simulink model "Assignment1_final"  (R2021a)
settings: Solver=FixedStepAuto  StartTime=0.0  StopTime=10.0  FixedStep=1e-3  RelTol=1e-3  EnableMultiTasking=on
undefined symbols (not defined in the file): a, b, c, D0, D1, D10, D11, D12, D13, D2, D3, D4, D5, D6, D7, D8, D9, magnitude, PTA0, PTA1, PTA2, PTB23, PTB9, PTC16, PTC17, PTC2, PTC3, PTC4, PTD0, PTD1, PTD2, PTD3
libraries: frdmk64flib x19, dspstat3 x1, hdlsllib x1
settings Model: EnablePacing=on  PacingRate=0.250000  ExtModeTrigDuration=5  Creator=Arun Mistry  LastModifiedBy=jesti
settings OptimizationCC: EnhancedBackFolding=on  PassReuseOutputArgsAs=Individual arguments  ZeroExternalMemoryAtStartup=off  ZeroInternalMemoryAtStartup=off  MaxStackSize=64  OptimizeBlockOrder=speed  DifferentSizesBufferReuse=on  OptimizationCustomize=off  EfficientTunableParamExpr=on
settings DebuggingCC: ParameterTunabilityLossMsg=error
settings HardwareCC: ProdBitPerPointer=32  ProdBitPerSizeT=32  ProdBitPerPtrDiffT=32  ProdLargestAtomicInteger=Long  ProdLargestAtomicFloat=Double  ProdWordSize=32  ProdHWDeviceType=ARM Compatible->ARM Cortex
settings SFSimCC: MATLABDynamicMemAlloc=off
settings RTWCC: SystemTargetFile=ert.tlc  HardwareBoard=NXP FRDM-K64F  TLCOptions="-aInlineSetEventsForThisBaseRateFcn=TLC_FALSE -aSuppressMultiTaskScheduler=TLC_FALSE  -aRateBasedStepFcn=0"  TemplateMakefile=ert_default_tmf  Toolchain=GNU Tools for ARM Embedded Processors
settings CodeAppCC: ForceParamTrailComments=on  IgnoreCustomStorageClasses=off  OperatorAnnotations=on  SimulinkDataObjDesc=on  SFDataObjDesc=on  InsertBlockDesc=on
settings ERTTargetCC: ExtModeTransport=4  ExtModeMexFile=sendToCommService

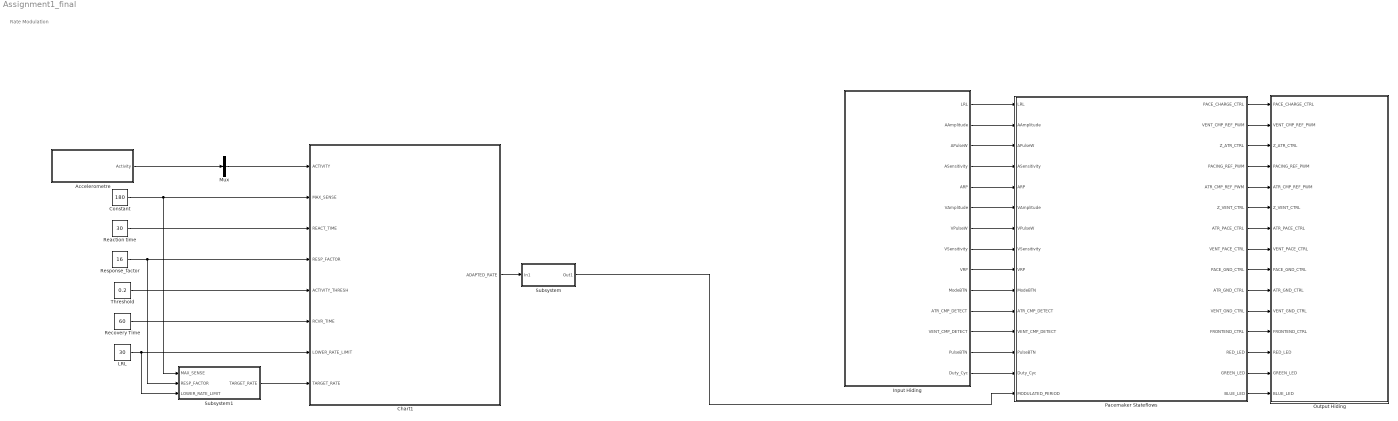
== system Assignment1_final ==
  note: Rate Modulation
  Accelerometre : Subsystem
  Chart1 : Stateflow chart  TreatAsAtomicUnit=on
  Constant : Constant  Value=180  OutDataTypeStr=uint16
  Input Hiding : Subsystem
  LRL : Constant  Value=30  OutDataTypeStr=uint16
  Mux : Mux  Inputs=1
  Output Hiding : Subsystem
  Pacemaker Stateflows : Stateflow chart  TreatAsAtomicUnit=on
      settings: PortSchema="{\"entries\":[{\"content\":{\"sides\":[{\"content\":{\"connectorIds\":[\"In1\",\"In2\",\"In3\",\"In4\",\"In5\",\"In6\",\"In7\",\"In8\",\"In9\",\"In10\",\"In11\",\"In12\",\"In13\",\"In15\",\"In14\"]},\"type\":\"ConnectorPlacement.EquallySpacedRectSide\",\"uuid\":\"73ec282f-bdc5-469f-8e6f-a94c3bdc9020\"},{\"content\":{\"connectorIds\":[\"Out1\",\"Out2\",\"Out3\",\"Out4\",\"Out5\",\"Out6\",\"Out7\",\"Out8\",\"Out9\",\"Out10\",\"Out11\",\"Out12\",\"Out13\",\"Out14\",\"Out15\"],\"side\":\"RIGHT\"},\"type\":\"ConnectorPlacement.EquallySpacedRectSide\",\"uuid\":\"8dd20006-a4c5-4baa-83a8-987332cd4bb4\"},{\"content\":{\"connectorIds\":[],\"side\":\"TOP\"},\"type\":\"ConnectorPlacement.EquallySpacedRectSide\",\"uuid\":\"22935e9b-efaa-43e1-8cc8-2e08fa14d9a6\"},{\"content\":{\"connectorIds\":[],\"side\":\"BOTTOM\"},\"type\":\"ConnectorPlacement.EquallySpacedRectSide\",\"uuid\":\"9851d334-d076-4ac0-89c9-77644970121a\"}]},\"type\":\"ConnectorPlacement.EquallySpacedConnector\",\"uuid\":\"2847227f-03fa-454f-95d6-41e472bd469d\"}],\"packageUris\":[\"http://schema.mathworks.com/mf0/Connector/R2020b\"],\"version\":\"1.0\"}"
  Reaction time : Constant  Value=30  OutDataTypeStr=uint16
  Recovery Time : Constant  Value=60  OutDataTypeStr=uint16
  Response_factor : Constant  Value=16  OutDataTypeStr=uint16
  Subsystem : Subsystem
  Subsystem1 : Subsystem
  Threshold : Constant  Value=0.2  OutDataTypeStr=double
  wires:
  Input Hiding/13(PulseBTN) -> Pacemaker Stateflows/13(PulseBTN)
  Pacemaker Stateflows/1(PACE_CHARGE_CTRL) -> Output Hiding/1(PACE_CHARGE_CTRL)
  Input Hiding/11(ATR_CMP_DETECT) -> Pacemaker Stateflows/11(ATR_CMP_DETECT)
  Input Hiding/7(VPulseW) -> Pacemaker Stateflows/7(VPulseW)
  Input Hiding/12(VENT_CMP_DETECT) -> Pacemaker Stateflows/12(VENT_CMP_DETECT)
  Pacemaker Stateflows/3(Z_ATR_CTRL) -> Output Hiding/3(Z_ATR_CTRL)
  Input Hiding/3(APulseW) -> Pacemaker Stateflows/3(APulseW)
  Pacemaker Stateflows/7(ATR_PACE_CTRL) -> Output Hiding/7(ATR_PACE_CTRL)
  Pacemaker Stateflows/10(ATR_GND_CTRL) -> Output Hiding/10(ATR_GND_CTRL)
  Input Hiding/10(ModeBTN) -> Pacemaker Stateflows/10(ModeBTN)
  Input Hiding/2(AAmplitude) -> Pacemaker Stateflows/2(AAmplitude)
  Input Hiding/6(VAmplitude) -> Pacemaker Stateflows/6(VAmplitude)
  Pacemaker Stateflows/6(Z_VENT_CTRL) -> Output Hiding/6(Z_VENT_CTRL)
  Pacemaker Stateflows/4(PACING_REF_PWM) -> Output Hiding/4(PACING_REF_PWM)
  Pacemaker Stateflows/11(VENT_GND_CTRL) -> Output Hiding/11(VENT_GND_CTRL)
  Pacemaker Stateflows/9(PACE_GND_CTRL) -> Output Hiding/9(PACE_GND_CTRL)
  Pacemaker Stateflows/8(VENT_PACE_CTRL) -> Output Hiding/8(VENT_PACE_CTRL)
  Input Hiding/1(LRL) -> Pacemaker Stateflows/1(LRL)
  Pacemaker Stateflows/15(BLUE_LED) -> Output Hiding/15(BLUE_LED)
  Input Hiding/4(ASensitivity) -> Pacemaker Stateflows/4(ASensitivity)
  Pacemaker Stateflows/12(FRONTEND_CTRL) -> Output Hiding/12(FRONTEND_CTRL)
  Input Hiding/9(VRP) -> Pacemaker Stateflows/9(VRP)
  Input Hiding/8(VSensitivity) -> Pacemaker Stateflows/8(VSensitivity)
  Input Hiding/5(ARP) -> Pacemaker Stateflows/5(ARP)
  Pacemaker Stateflows/14(GREEN_LED) -> Output Hiding/14(GREEN_LED)
  Pacemaker Stateflows/13(RED_LED) -> Output Hiding/13(RED_LED)
  Pacemaker Stateflows/5(ATR_CMP_REF_PWM) -> Output Hiding/5(ATR_CMP_REF_PWM)
  Pacemaker Stateflows/2(VENT_CMP_REF_PWM) -> Output Hiding/2(VENT_CMP_REF_PWM)
  Input Hiding/14(Duty_Cyc) -> Pacemaker Stateflows/15(Duty_Cyc)
  LRL/1 -> Chart1/7(LOWER_RATE_LIMIT), Subsystem1/3(LOWER_RATE_LIMIT)
  Chart1/1(ADAPTED_RATE) -> Subsystem/1(In1)
  Subsystem1/1(TARGET_RATE) -> Chart1/8(TARGET_RATE)
  Mux/1 -> Chart1/1(ACTIVITY)
  Recovery Time/1 -> Chart1/6(RCVR_TIME)
  Constant/1 -> Subsystem1/1(MAX_SENSE), Chart1/2(MAX_SENSE)
  Reaction time/1 -> Chart1/3(REACT_TIME)
  Response_factor/1 -> Subsystem1/2(RESP_FACTOR), Chart1/4(RESP_FACTOR)
  Accelerometre/1(Activity) -> Mux/1
  Threshold/1 -> Chart1/5(ACTIVITY_THRESH)
  Subsystem/1(Out1) -> Pacemaker Stateflows/14(MODULATED_PERIOD)

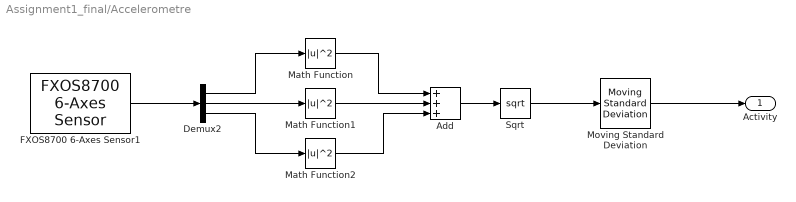
== system Assignment1_final/Accelerometre ==
  Add : Sum  Inputs=+++
  Demux2 : Demux  Outputs=3
  FXOS8700 6-Axes Sensor1 : frdmk64flib/FXOS8700 6-Axes Sensor  Activesensor=Accelerometer only  ODR=800Hz  HybridODR=400Hz  Accelfullrange=-4g to +4g  SampleTime=-1
  Math Function : Math  Operator=magnitude^2  SignedPower=on  OutDataTypeStr=double  SaturateOnIntegerOverflow=on
  Math Function1 : Math  Operator=magnitude^2  SignedPower=on  OutDataTypeStr=double  SaturateOnIntegerOverflow=on
  Math Function2 : Math  Operator=magnitude^2  SignedPower=on  OutDataTypeStr=double  SaturateOnIntegerOverflow=on
  Moving Standard Deviation : dspstat3/Moving Standard Deviation  Method=Sliding window  ForgettingFactorPort=off  SpecifyWindowLength=on  WindowLength=128  ForgettingFactor=0.9  SimulateUsing=Code generation
      settings: SourceProductBaseCode=DS
  Sqrt : Sqrt  SaturateOnIntegerOverflow=on
  Activity : Outport  SourceOfInitialOutputValue=Input signal
  wires:
  Sqrt/1 -> Moving Standard Deviation/1
  FXOS8700 6-Axes Sensor1/1 -> Demux2/1
  Math Function/1 -> Add/1
  Add/1 -> Sqrt/1
  Math Function2/1 -> Add/3
  Demux2/2 -> Math Function1/1
  Math Function1/1 -> Add/2
  Demux2/1 -> Math Function/1
  Demux2/3 -> Math Function2/1
  Moving Standard Deviation/1 -> Activity/1

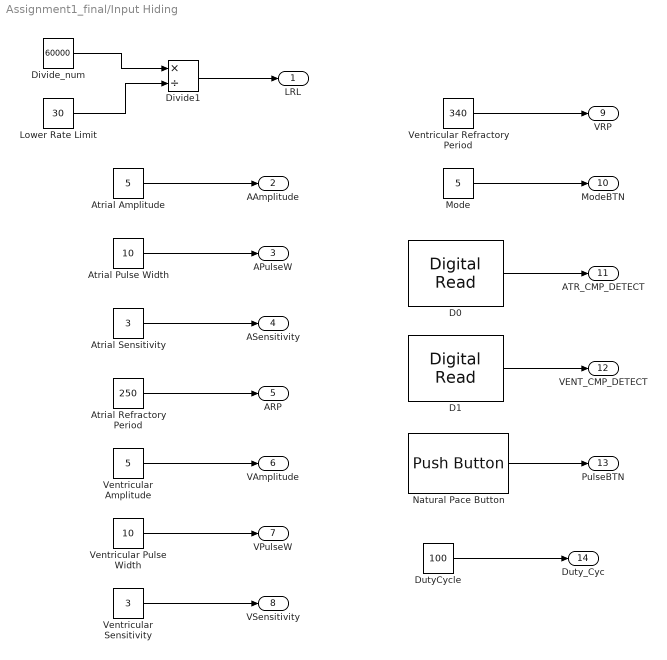
== system Assignment1_final/Input Hiding ==
  Atrial Amplitude : Constant  Value=5  OutDataTypeStr=uint16
  Atrial Pulse Width : Constant  Value=10  OutDataTypeStr=uint16
  Atrial Refractory Period : Constant  Value=250  OutDataTypeStr=uint16
  Atrial Sensitivity : Constant  Value=3  OutDataTypeStr=uint16
  D0 : frdmk64flib/Digital Read  Whichpin=PTC16 (D0)  SampleTime=-1
  D1 : frdmk64flib/Digital Read  Whichpin=PTC17 (D1)  SampleTime=-1
  Divide1 : Product  Inputs=*/  OutDataTypeStr=uint16  RndMeth=Round
  Divide_num : Constant  Value=60000  OutDataTypeStr=uint16
  DutyCycle : Constant  Value=100  OutDataTypeStr=uint16
  Lower Rate Limit : Constant  Value=30  OutDataTypeStr=uint16
  Mode : Constant  Value=5  OutDataTypeStr=uint16
  Natural Pace Button : frdmk64flib/Push Button  Whichswitch=SW3  SampleTime1=-1
  Ventricular Amplitude : Constant  Value=5  OutDataTypeStr=uint16
  Ventricular Pulse Width : Constant  Value=10  OutDataTypeStr=uint16
  Ventricular Refractory Period : Constant  Value=340  OutDataTypeStr=uint16
  Ventricular Sensitivity : Constant  Value=3  OutDataTypeStr=uint16
  LRL : Outport  OutDataTypeStr=uint16
  AAmplitude : Outport  Port=2  OutDataTypeStr=uint16
  APulseW : Outport  Port=3  OutDataTypeStr=uint16
  ASensitivity : Outport  Port=4  OutDataTypeStr=uint16
  ARP : Outport  Port=5  OutDataTypeStr=uint16
  VAmplitude : Outport  Port=6  OutDataTypeStr=uint16
  VPulseW : Outport  Port=7  OutDataTypeStr=uint16
  VSensitivity : Outport  Port=8  OutDataTypeStr=uint16
  VRP : Outport  Port=9  OutDataTypeStr=uint16
  ModeBTN : Outport  Port=10  OutDataTypeStr=uint16
  ATR_CMP_DETECT : Outport  Port=11  OutDataTypeStr=boolean
  VENT_CMP_DETECT : Outport  Port=12  OutDataTypeStr=boolean
  PulseBTN : Outport  Port=13  OutDataTypeStr=boolean
  Duty_Cyc : Outport  Port=14  OutDataTypeStr=uint16
  wires:
  Atrial Amplitude/1 -> AAmplitude/1
  Ventricular Amplitude/1 -> VAmplitude/1
  Atrial Pulse Width/1 -> APulseW/1
  Ventricular Pulse Width/1 -> VPulseW/1
  Atrial Sensitivity/1 -> ASensitivity/1
  Ventricular Sensitivity/1 -> VSensitivity/1
  Ventricular Refractory Period/1 -> VRP/1
  Atrial Refractory Period/1 -> ARP/1
  D1/1 -> VENT_CMP_DETECT/1
  D0/1 -> ATR_CMP_DETECT/1
  Natural Pace Button/1 -> PulseBTN/1
  Mode/1 -> ModeBTN/1
  DutyCycle/1 -> Duty_Cyc/1
  Lower Rate Limit/1 -> Divide1/2
  Divide_num/1 -> Divide1/1
  Divide1/1 -> LRL/1

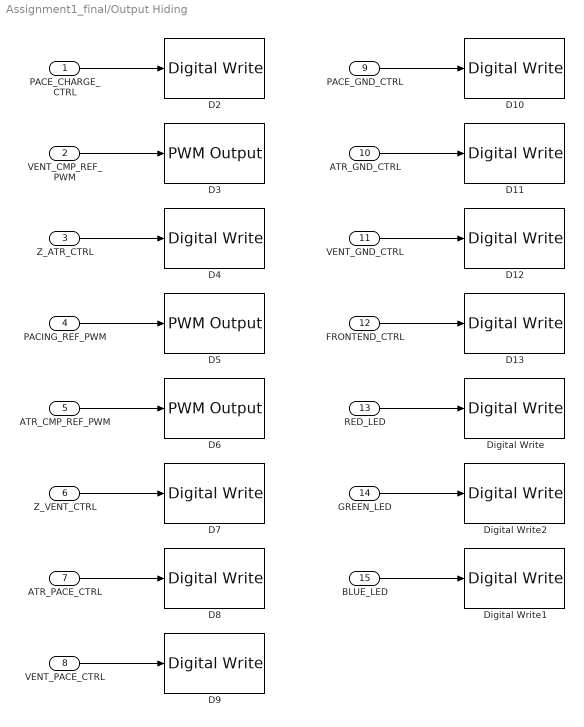
== system Assignment1_final/Output Hiding ==
  PACE_CHARGE_CTRL : Inport  OutDataTypeStr=uint16
  VENT_CMP_REF_PWM : Inport  Port=2  OutDataTypeStr=uint16
  Z_ATR_CTRL : Inport  Port=3  OutDataTypeStr=uint16
  PACING_REF_PWM : Inport  Port=4  OutDataTypeStr=uint16
  ATR_CMP_REF_PWM : Inport  Port=5  OutDataTypeStr=uint16
  Z_VENT_CTRL : Inport  Port=6  OutDataTypeStr=uint16
  ATR_PACE_CTRL : Inport  Port=7  OutDataTypeStr=uint16
  VENT_PACE_CTRL : Inport  Port=8  OutDataTypeStr=uint16
  PACE_GND_CTRL : Inport  Port=9  OutDataTypeStr=uint16
  ATR_GND_CTRL : Inport  Port=10  OutDataTypeStr=uint16
  VENT_GND_CTRL : Inport  Port=11  OutDataTypeStr=uint16
  FRONTEND_CTRL : Inport  Port=12  OutDataTypeStr=uint16
  RED_LED : Inport  Port=13  OutDataTypeStr=uint16
  GREEN_LED : Inport  Port=14  OutDataTypeStr=uint16
  BLUE_LED : Inport  Port=15  OutDataTypeStr=uint16
  D10 : frdmk64flib/Digital Write  Whichpin=PTD0 (D10)
  D11 : frdmk64flib/Digital Write  Whichpin=PTD2 (D11)
  D12 : frdmk64flib/Digital Write  Whichpin=PTD3 (D12)
  D13 : frdmk64flib/Digital Write  Whichpin=PTD1 (D13)
  D2 : frdmk64flib/Digital Write  Whichpin=PTB9 (D2)
  D3 : frdmk64flib/PWM Output  Whichpin=PTA1 (D3)  InitialFrequency=2000  InitialDutyCycle=100
  D4 : frdmk64flib/Digital Write  Whichpin=PTB23 (D4)
  D5 : frdmk64flib/PWM Output  Whichpin=PTA2 (D5)  InitialFrequency=2000  InitialDutyCycle=100
  D6 : frdmk64flib/PWM Output  Whichpin=PTC2 (D6)  InitialFrequency=2000  InitialDutyCycle=100
  D7 : frdmk64flib/Digital Write  Whichpin=PTC3 (D7)
  "D8 " : frdmk64flib/Digital Write  Whichpin=PTA0 (D8)
  D9 : frdmk64flib/Digital Write  Whichpin=PTC4 (D9)
  Digital Write : frdmk64flib/Digital Write  Whichpin=RED_LED
  Digital Write1 : frdmk64flib/Digital Write  Whichpin=BLUE_LED
  Digital Write2 : frdmk64flib/Digital Write  Whichpin=GREEN_LED
  wires:
  VENT_PACE_CTRL/1 -> D9/1
  ATR_CMP_REF_PWM/1 -> D6/1
  PACE_GND_CTRL/1 -> D10/1
  VENT_CMP_REF_PWM/1 -> D3/1
  PACING_REF_PWM/1 -> D5/1
  ATR_GND_CTRL/1 -> D11/1
  ATR_PACE_CTRL/1 -> "D8 "/1
  PACE_CHARGE_CTRL/1 -> D2/1
  FRONTEND_CTRL/1 -> D13/1
  VENT_GND_CTRL/1 -> D12/1
  Z_ATR_CTRL/1 -> D4/1
  Z_VENT_CTRL/1 -> D7/1
  RED_LED/1 -> Digital Write/1
  BLUE_LED/1 -> Digital Write1/1
  GREEN_LED/1 -> Digital Write2/1

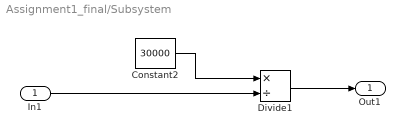
== system Assignment1_final/Subsystem ==
  In1 : Inport  OutDataTypeStr=uint16
  Constant2 : Constant  Value=30000  OutDataTypeStr=uint16
  Divide1 : Product  Inputs=*/  OutDataTypeStr=uint16
  Out1 : Outport  OutDataTypeStr=uint16
  wires:
  In1/1 -> Divide1/2
  Constant2/1 -> Divide1/1
  Divide1/1 -> Out1/1

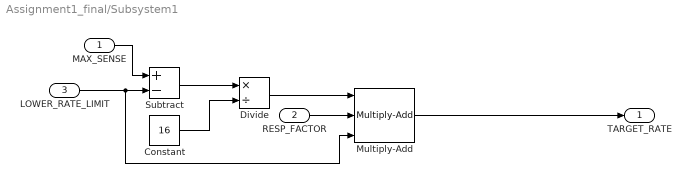
== system Assignment1_final/Subsystem1 ==
  MAX_SENSE : Inport  OutDataTypeStr=uint16
  RESP_FACTOR : Inport  Port=2  OutDataTypeStr=uint16
  LOWER_RATE_LIMIT : Inport  Port=3  OutDataTypeStr=uint16
  Constant : Constant  Value=16  OutDataTypeStr=uint16
  Divide : Product  Inputs=*/  OutDataTypeStr=uint16
  Multiply-Add : hdlsllib/HDL Operations/Multiply-Add  Function=c+(a.*b)  datatype=uint16  RndMeth=Nearest  DoSatur=off  FMA=off
      settings: SourceProductBaseCode=SL
  Subtract : Sum  Inputs=+-  AccumDataTypeStr=uint16
  TARGET_RATE : Outport  OutDataTypeStr=uint16  SourceOfInitialOutputValue=Input signal
  wires:
  MAX_SENSE/1 -> Subtract/1
  LOWER_RATE_LIMIT/1 -> Multiply-Add/3, Subtract/2
  Subtract/1 -> Divide/1
  Constant/1 -> Divide/2
  Divide/1 -> Multiply-Add/1
  RESP_FACTOR/1 -> Multiply-Add/2
  Multiply-Add/1 -> TARGET_RATE/1

== stateflow chart Assignment1_final/Pacemaker Stateflows ==
  state MODE_CHOOSE
  state AOO
    entry:
    VENT_PACE_CTRL = 0; VENT_GND_CTRL = 0; PACE_GND_CTRL = 1; Z_VENT_CTRL = 0;
    Z_ATR_CTRL = 0;ATR_PACE_CTRL = 0; PACING_REF_PWM = Duty_Cyc;
    state PACE_ATR
      entry:
      PACE_CHARGE_CTRL = 0;
      ATR_GND_CTRL = 0;
      ATR_PACE_CTRL = 1;
      RED_LED = 1;
    state C22_CHARGE
      entry:
      PACE_CHARGE_CTRL = 1;
      ATR_PACE_CTRL = 0;
      ATR_GND_CTRL = 1;
      RED_LED = 0;
    (default) -> AOO.C22_CHARGE
    AOO.PACE_ATR -> AOO.C22_CHARGE : after(APulseW,msec)
    AOO.C22_CHARGE -> AOO.PACE_ATR : after(LRL-APulseW,msec)
  state VOO
    entry:
    ATR_PACE_CTRL = 0; ATR_GND_CTRL = 0; PACE_GND_CTRL = 1;
    Z_ATR_CTRL = 0; Z_VENT_CTRL = 0; PACING_REF_PWM = Duty_Cyc;
    state PACE_VENT
      entry:
      PACE_CHARGE_CTRL = 0;
      VENT_GND_CTRL = 0;
      VENT_PACE_CTRL = 1;
      BLUE_LED = 1;
    state C22_CHARGE
      entry:
      VENT_PACE_CTRL = 0;
      VENT_GND_CTRL = 1;
      PACE_CHARGE_CTRL = 1;
      BLUE_LED = 0;
    (default) -> VOO.C22_CHARGE
    VOO.PACE_VENT -> VOO.C22_CHARGE : after(VPulseW,msec)
    VOO.C22_CHARGE -> VOO.PACE_VENT : after(LRL-VPulseW,msec)
  state AAI
    entry:
    VENT_PACE_CTRL = 0; VENT_GND_CTRL = 0; ATR_CMP_REF_PWM=(ASensitivity/AAmplitude)*100;
    Z_VENT_CTRL = 0; Z_ATR_CTRL = 0;PACING_REF_PWM = Duty_Cyc;PACE_GND_CTRL = 1;FRONTEND_CTRL = 1; sense = 0;pace=0;
    state C22_CHARGE
      entry:
      RED_LED = 0;
      PACE_CHARGE_CTRL = 1;
      ATR_GND_CTRL = 1;
      ATR_PACE_CTRL = 0;
      sense = 0;
    state PACE_ATR
      entry:
      RED_LED = 1;
      PACE_CHARGE_CTRL = 0;
      ATR_GND_CTRL = 0;
      ATR_PACE_CTRL = 1;
      sense = 1;pace=1;
    state REFRACTORY
      entry:
      GREEN_LED = 1;
      PACE_CHARGE_CTRL = 1;
      ATR_GND_CTRL = 1;
      ATR_PACE_CTRL = 0;
    (default) -> AAI.C22_CHARGE
    AAI.REFRACTORY -> AAI.C22_CHARGE : after(ARP-(APulseW * sense),msec)
    AAI.C22_CHARGE -> AAI.PACE_ATR [order 2] : after(LRL-ARP,msec)
    AAI.PACE_ATR -> AAI.REFRACTORY : after(APulseW,msec)
    AAI.C22_CHARGE -> AAI.REFRACTORY [order 1] : [ATR_CMP_DETECT == true && pace==1]
  state VVI
    entry:
    ATR_PACE_CTRL = 0; ATR_GND_CTRL = 0; PACE_GND_CTRL = 1; VENT_CMP_REF_PWM=(VSensitivity/VAmplitude)*100
    Z_VENT_CTRL = 0; Z_ATR_CTRL = 0;FRONTEND_CTRL = 1; PACING_REF_PWM = Duty_Cyc; pace = 0; sense = 0;
    state PACE_VENT
      entry:
      BLUE_LED = 1;
      PACE_CHARGE_CTRL = 0;
      VENT_GND_CTRL = 0;
      VENT_PACE_CTRL = 1;
      pace = 1; sense = 1
    state C22_CHARGE
      entry:
      BLUE_LED = 0;
      PACE_CHARGE_CTRL = 1;
      VENT_GND_CTRL = 1;
      VENT_PACE_CTRL = 0;
      sense = 0;
    state REFRACTORY
      entry:
      GREEN_LED = 1;
      PACE_CHARGE_CTRL = 1;
      VENT_GND_CTRL = 1;
      VENT_PACE_CTRL = 0;
    (default) -> VVI.C22_CHARGE
    VVI.C22_CHARGE -> VVI.PACE_VENT [order 2] : after(LRL-VRP,msec)
    VVI.REFRACTORY -> VVI.C22_CHARGE : after(VRP-(VPulseW *sense),msec)
    VVI.PACE_VENT -> VVI.REFRACTORY : after(VPulseW,msec)
    VVI.C22_CHARGE -> VVI.REFRACTORY [order 1] : [VENT_CMP_DETECT == true && pace==1]
  state AOOR
    entry:
    VENT_PACE_CTRL = 0; VENT_GND_CTRL = 0; ATR_CMP_REF_PWM=(ASensitivity/AAmplitude)*100;
    Z_VENT_CTRL = 0; Z_ATR_CTRL = 0;PACING_REF_PWM = Duty_Cyc;PACE_GND_CTRL = 1;FRONTEND_CTRL = 1; sense = 0;pace=0;
    state CHARGING
      during:
      %Begin Charging C22 Capacitor
      ATR_PACE_CTRL = 0
      VENT_PACE_CTRL = 0
      PACING_REF_PWM = Duty_Cyc
      PACE_CHARGE_CTRL = 1
      %Begin Discharging C21 Blocking Capacitor
      PACE_GND_CTRL = 1
      VENT_PACE_CTRL = 0
      Z_ATR_CTRL = 0
      Z_VENT_CTRL = 0
      ATR_PACE_CTRL = 0
      ATR_GND_CTRL = 1
      VENT_GND_CTRL = 0
    state DISCHARGING
      during:
      %Discharge C22 into Atrium (AtrialPacing)
      %Begin Charging C21 Blocking Capacitor
      PACE_CHARGE_CTRL = 0
      PACE_GND_CTRL = 1
      ATR_PACE_CTRL = 1
      ATR_GND_CTRL = 0
      Z_ATR_CTRL = 0
      Z_VENT_CTRL = 0
      VENT_GND_CTRL = 0
      VENT_PACE_CTRL  = 0
    (default) -> AOOR.CHARGING
    AOOR.CHARGING -> AOOR.DISCHARGING : after(MODULATED_PERIOD - APulseW, msec)
    AOOR.DISCHARGING -> AOOR.CHARGING : after(APulseW, msec)
  state VOOR [commented out]
    state CHARGING [commented out]
      during:
      %Begin Charging C22 Capacitor
      ATR_PACE_CTRL = LOW
      VENT_PACE_CTRL = LOW
      PACING_REF_PWM = Duty_Cyc;
      PACE_CHARGE_CTRL = HIGH
      %Begin Discharging C21 Blocking Capacitor
      PACE_GND_CTRL = HIGH
      VENT_PACE_CTRL = LOW
      Z_ATR_CTRL = LOW
      Z_VENT_CTRL = LOW
      ATR_PACE_CTRL = LOW
      ATR_GND_CTRL = LOW
      VENT_GND_CTRL = HIGH
    state DISCHARGING [commented out]
      during:
      %Discharge C22 into Ventricle (Vent Pacing)
      %Begin Charging Blocking Capacitor
      PACE_CHARGE_CTRL = LOW
      PACE_GND_CTRL = HIGH
      ATR_PACE_CTRL = LOW
      ATR_GND_CTRL = LOW
      Z_ATR_CTRL = LOW
      Z_VENT_CTRL = LOW
      VENT_GND_CTRL = LOW
      VENT_PACE_CTRL  = HIGH
    (default) -> VOOR.CHARGING [commented out]
    VOOR.CHARGING -> VOOR.DISCHARGING [commented out] : after(MODULATED_PERIOD - VPulseW, msec)
    VOOR.DISCHARGING -> VOOR.CHARGING [commented out] : after(VPulseW,msec)
  state DOO [commented out]
    state ATR_CHARGING [commented out]
      during:
      %Begin Charging C22 Capacitor
      ATR_PACE_CTRL = LOW
      VENT_PACE_CTRL = LOW
      PACING_REF_PWM = ATR_DUTY_CYCLE
      PACE_CHARGE_CTRL = HIGH
      %Begin Discharging C21 Blocking Capacitor
      PACE_GND_CTRL = HIGH
      VENT_PACE_CTRL = LOW
      Z_ATR_CTRL = LOW
      Z_VENT_CTRL = LOW
      ATR_PACE_CTRL = LOW
      ATR_GND_CTRL = HIGH
      VENT_GND_CTRL = LOW
    state VENT_CHARGING [commented out]
      during:
      %Begin Charging C22 Capacitor
      ATR_PACE_CTRL = LOW
      VENT_PACE_CTRL = LOW
      PACING_REF_PWM = VENT_DUTY_CYCLE
      PACE_CHARGE_CTRL = HIGH
      %Begin Discharging C21 Blocking Capacitor
      PACE_GND_CTRL = HIGH
      VENT_PACE_CTRL = LOW
      Z_ATR_CTRL = LOW
      Z_VENT_CTRL = LOW
      ATR_PACE_CTRL = LOW
      ATR_GND_CTRL = LOW
      VENT_GND_CTRL = HIGH
    state ATR_DISCHARGING [commented out]
      during:
      %Discharge C22 into Atrium (AtrialPacing)
      %Begin Charging C21 Blocking Capacitor
      PACE_CHARGE_CTRL = LOW
      PACE_GND_CTRL = HIGH
      ATR_PACE_CTRL = HIGH
      ATR_GND_CTRL = LOW
      Z_ATR_CTRL = LOW
      Z_VENT_CTRL = LOW
      VENT_GND_CTRL = LOW
      VENT_PACE_CTRL  = LOW
    state VENT_DISCHARGING [commented out]
      during:
      %Discharge C22 into Ventricle (Vent Pacing)
      %Begin Charging Blocking Capacitor
      PACE_CHARGE_CTRL = LOW
      PACE_GND_CTRL = HIGH
      ATR_PACE_CTRL = LOW
      ATR_GND_CTRL = LOW
      Z_ATR_CTRL = LOW
      Z_VENT_CTRL = LOW
      VENT_GND_CTRL = LOW
      VENT_PACE_CTRL  = HIGH
    VENT_DISCHARGING -> VENT_CHARGING [commented out] : after(VPulseW,msec)
    DOO -> VENT_CHARGING [commented out] : [MODE == 5]
    ATR_DISCHARGING -> ATR_CHARGING [commented out] : after(APulseW, msec)
    ATR_CHARGING -> VENT_DISCHARGING [commented out] : after(0.15 - APulseW,msec)
    VENT_CHARGING -> ATR_DISCHARGING [commented out] : after(LRL/60000 - VPulseW - 0.15, msec)
    VENT_CHARGING -> DOO [commented out] : [MODE ~= 5]
  state DOOR [commented out]
    state ATR_CHARGING1 [commented out]
      during:
      %Begin Charging C22 Capacitor
      ATR_PACE_CTRL = LOW
      VENT_PACE_CTRL = LOW
      PACING_REF_PWM = ATR_DUTY_CYCLE
      PACE_CHARGE_CTRL = HIGH
      %Begin Discharging C21 Blocking Capacitor
      PACE_GND_CTRL = HIGH
      VENT_PACE_CTRL = LOW
      Z_ATR_CTRL = LOW
      Z_VENT_CTRL = LOW
      ATR_PACE_CTRL = LOW
      ATR_GND_CTRL = HIGH
      VENT_GND_CTRL = LOW
    state VENT_CHARGING1 [commented out]
      during:
      %Begin Charging C22 Capacitor
      ATR_PACE_CTRL = LOW
      VENT_PACE_CTRL = LOW
      PACING_REF_PWM = VENT_DUTY_CYCLE
      PACE_CHARGE_CTRL = HIGH
      %Begin Discharging C21 Blocking Capacitor
      PACE_GND_CTRL = HIGH
      VENT_PACE_CTRL = LOW
      Z_ATR_CTRL = LOW
      Z_VENT_CTRL = LOW
      ATR_PACE_CTRL = LOW
      ATR_GND_CTRL = LOW
      VENT_GND_CTRL = HIGH
    state ATR_DISCHARGING1 [commented out]
      during:
      %Discharge C22 into Atrium (AtrialPacing)
      %Begin Charging C21 Blocking Capacitor
      PACE_CHARGE_CTRL = LOW
      PACE_GND_CTRL = HIGH
      ATR_PACE_CTRL = HIGH
      ATR_GND_CTRL = LOW
      Z_ATR_CTRL = LOW
      Z_VENT_CTRL = LOW
      VENT_GND_CTRL = LOW
      VENT_PACE_CTRL  = LOW
    state VENT_DISCHARGING1 [commented out]
      during:
      %Discharge C22 into Ventricle (Vent Pacing)
      %Begin Charging Blocking Capacitor
      PACE_CHARGE_CTRL = LOW
      PACE_GND_CTRL = HIGH
      ATR_PACE_CTRL = LOW
      ATR_GND_CTRL = LOW
      Z_ATR_CTRL = LOW
      Z_VENT_CTRL = LOW
      VENT_GND_CTRL = LOW
      VENT_PACE_CTRL  = HIGH
    VENT_DISCHARGING1 -> VENT_CHARGING1 [commented out] : after(VPulseW,msec)
    DOOR -> VENT_CHARGING1 [commented out] : [MODE == 6]
    ATR_DISCHARGING1 -> ATR_CHARGING1 [commented out] : after(APulseW, msec)
    ATR_CHARGING1 -> VENT_DISCHARGING1 [commented out] : after(0.15-VPulseW,msec)
    VENT_CHARGING1 -> ATR_DISCHARGING1 [commented out] : after(MODULATED_PERIOD - VPulseW - 0.15, msec)
    VENT_CHARGING1 -> DOOR [commented out] : [MODE ~= 6]
  state AAIR [commented out]
    state PROXY [commented out]
      during:
      %Discharge C21 Blocking Capacitor
      PACE_GND_CTRL = HIGH
      VENT_PACE_CTRL = LOW
      Z_ATR_CTRL = LOW
      Z_VENT_CTRL = LOW
      ATR_PACE_CTRL = LOW
      ATR_GND_CTRL = HIGH
      VENT_GND_CTRL = LOW
      %Charge C22
      ATR_PACE_CTRL = LOW
      VENT_PACE_CTRL = LOW
      PACING_REF_PWM = ATR_DUTY_CYCLE
      PACE_CHARGE_CTRL = HIGH
    state DISCHARGING [commented out]
      during:
      %Discharge C22 into Atrium (Atrial Pacing)
      %Begin Charging Blocking Capacitor
      PACE_CHARGE_CTRL = LOW
      PACE_GND_CTRL = HIGH
      ATR_PACE_CTRL = HIGH
      ATR_GND_CTRL = LOW
      Z_ATR_CTRL = LOW
      Z_VENT_CTRL = LOW
      VENT_GND_CTRL = LOW
      VENT_PACE_CTRL  = LOW
    state CHARGING [commented out]
      during:
      %Begin Charging C22 Capacitor
      ATR_PACE_CTRL = LOW
      VENT_PACE_CTRL = LOW
      PACING_REF_PWM = ATR_DUTY_CYCLE
      PACE_CHARGE_CTRL = HIGH
      %Begin Discharging C21 Blocking Capacitor
      PACE_GND_CTRL = HIGH
      VENT_PACE_CTRL = LOW
      Z_ATR_CTRL = LOW
      Z_VENT_CTRL = LOW
      ATR_PACE_CTRL = LOW
      ATR_GND_CTRL = HIGH
      VENT_GND_CTRL = LOW
    AAIR.DISCHARGING -> AAIR.PROXY [commented out] : after(APulseW,msec)
    AAIR.PROXY -> AAIR.CHARGING [commented out] : after(ARP, msec)
    (junction 521) -> AAIR.PROXY [commented out] : after(LRL,msec)
    AAIR -> AAIR.CHARGING [commented out] : [MODE == 9]
    AAIR.CHARGING -> (junction 521) [commented out] : [ATR_CMP_DETECT == HIGH]
    AAIR.CHARGING -> AAIR.DISCHARGING [commented out] : after(MODULATED_PERIOD - APulseW-ARP,msec)
    AAIR.CHARGING -> AAIR [commented out] : [MODE ~= 9]
  state VVIR [commented out]
    state PROXY [commented out]
      during:
      %Step 1
      %Discharge C21 Blocking Capacitor
      PACE_GND_CTRL = HIGH
      VENT_PACE_CTRL = LOW
      Z_ATR_CTRL = LOW
      Z_VENT_CTRL = LOW
      ATR_PACE_CTRL = LOW
      ATR_GND_CTRL = LOW
      VENT_GND_CTRL = HIGH
      %Step 2
      %Charge C22
      ATR_PACE_CTRL = LOW
      VENT_PACE_CTRL = LOW
      PACING_REF_PWM = VENT_DUTY_CYCLE
      PACE_CHARGE_CTRL = HIGH
    state CHARGING [commented out]
      during:
      %Begin Charging C22 Capacitor
      ATR_PACE_CTRL = LOW
      VENT_PACE_CTRL = LOW
      PACING_REF_PWM = VENT_DUTY_CYCLE
      PACE_CHARGE_CTRL = HIGH
      %Begin Discharging Blocking Capacitor
      PACE_GND_CTRL = HIGH
      VENT_PACE_CTRL = LOW
      Z_ATR_CTRL = LOW
      Z_VENT_CTRL = LOW
      ATR_PACE_CTRL = LOW
      ATR_GND_CTRL = LOW
      VENT_GND_CTRL = HIGH
    state DISCHARGING [commented out]
      during:
      %Step 1:
      %Discharge C22 into Ventricle (Vent Pacing)
      %Begin Charging Blocking Capacitor
      PACE_CHARGE_CTRL = LOW
      PACE_GND_CTRL = HIGH
      ATR_PACE_CTRL = LOW
      ATR_GND_CTRL = LOW
      Z_ATR_CTRL = LOW
      Z_VENT_CTRL = LOW
      VENT_GND_CTRL = LOW
      VENT_PACE_CTRL  = HIGH
    VVIR.DISCHARGING -> VVIR.PROXY [commented out] : after(VPulseW, msec)
    VVIR.PROXY -> VVIR.CHARGING [commented out] : after(VRP, msec)
    VVIR -> VVIR.CHARGING [commented out] : [MODE == 10]
    (junction 543) -> VVIR.PROXY [commented out] : after(LRL,msec)
    VVIR.CHARGING -> VVIR [commented out] : [MODE ~= 10]
    VVIR.CHARGING -> (junction 543) [commented out] : [VENT_CMP_DETECT ==  HIGH]
    VVIR.CHARGING -> VVIR.DISCHARGING [commented out] : after(MODULATED_PERIOD - VPulseW - VRP,msec)
  MODE_CHOOSE -> AOO [order 1] : [ModeBTN==1]
  (default) -> MODE_CHOOSE
  AOO -> MODE_CHOOSE : [ModeBTN~=1]
  MODE_CHOOSE -> VOO [order 2] : [ModeBTN==2]
  VOO -> MODE_CHOOSE : [ModeBTN~=2]
  MODE_CHOOSE -> AAI [order 4] : [ModeBTN==3]
  AAI -> MODE_CHOOSE : [ModeBTN~=3]
  MODE_CHOOSE -> VVI [order 5] : [ModeBTN==4]
  VVI -> MODE_CHOOSE : [ModeBTN~=4]
  MODE_CHOOSE -> AOOR [order 3] : [ModeBTN==5]
  AOOR -> MODE_CHOOSE : [ModeBTN~=5]
  MODE_CHOOSE -> VOOR [commented out] : [ModeBTN==6]
  VOOR -> MODE_CHOOSE [commented out] : [ModeBTN~=6]
  MODE_CHOOSE -> DOO [commented out] : [ModeBTN==5]
  DOO -> MODE_CHOOSE [commented out] : [ModeBTN~=5]
  MODE_CHOOSE -> DOOR [commented out] : [ModeBTN==6]
  DOOR -> MODE_CHOOSE [commented out] : [ModeBTN~=6]
  MODE_CHOOSE -> AAIR [commented out] : [ModeBTN==7]
  AAIR -> MODE_CHOOSE [commented out] : [ModeBTN~=7]
  MODE_CHOOSE -> VVIR [commented out] : [ModeBTN==8]
  VVIR -> MODE_CHOOSE [commented out] : [ModeBTN~=8]
  data: LRL input uint16; AAmplitude input uint16; APulseW input uint16; ASensitivity input uint16; ARP input uint16; VAmplitude input uint16; VPulseW input uint16; VSensitivity input uint16; VRP input uint16; PACE_CHARGE_CTRL output uint16; VENT_CMP_REF_PWM output uint16; Z_ATR_CTRL output uint16; PACING_REF_PWM output uint16; ATR_CMP_REF_PWM output uint16; Z_VENT_CTRL output uint16; ATR_PACE_CTRL output uint16; VENT_PACE_CTRL output uint16; PACE_GND_CTRL output uint16; ATR_GND_CTRL output uint16; VENT_GND_CTRL output uint16; ModeBTN input uint16; FRONTEND_CTRL output uint16; RED_LED output uint16; GREEN_LED output uint16; BLUE_LED output uint16; ATR_CMP_DETECT input boolean; VENT_CMP_DETECT input boolean; PulseBTN input boolean; MODULATED_PERIOD input uint16; Duty_Cyc input uint16; sense local uint16; pace local uint16

== stateflow chart Assignment1_final/Chart1 ==
  state Start [commented out]
    entry:
    ADAPTED_RATE = LOWER_RATE_LIMIT;
  state S1 [commented out]
    entry:
    ADAPTED_RATE = ADAPTED_RATE + step_up;
  state S4
    entry:
    ADAPTED_RATE = ADAPTED_RATE + step_up;
  state S2 [commented out]
    entry:
    ADAPTED_RATE = MAX_SENSE;
  state S3
    entry:
    ADAPTED_RATE = TARGET_RATE;
  state Start1
    entry:
    ADAPTED_RATE = LOWER_RATE_LIMIT;
  state S_FAILSAFE1
    entry:
    ADAPTED_RATE = ADAPTED_RATE - step_up;
  state S_FAILSAFE [commented out]
    entry:
  state S2FAIL [commented out]
    entry:
    ADAPTED_RATE = ADAPTED_RATE - step_down;
  state S2FAIL1
    entry:
    ADAPTED_RATE = ADAPTED_RATE - step_down;
  (default) -> Start [commented out] : {step_up = RESP_FACTOR * (MAX_SENSE - LOWER_RATE_LIMIT) / REACT_TIME,
      | step_down = RESP_FACTOR * (MAX_SENSE - LOWER_RATE_LIMIT)  / RCVR_TIME}
  (default) -> Start1 : {step_up = ceil((TARGET_RATE - LOWER_RATE_LIMIT) / REACT_TIME),
      | step_down = ceil((TARGET_RATE - LOWER_RATE_LIMIT)  / (RCVR_TIME))}
  S1 -> S1 [commented out] : after(1000,msec)[ADAPTED_RATE ~= MAX_SENSE]
  S4 -> S4 [order 1] : after(1000,msec)[ADAPTED_RATE <= TARGET_RATE]
  S2 -> S2 [commented out] : [ACTIVITY > ACTIVITY_THRESH]
  S3 -> S3 [order 2] : [ACTIVITY > ACTIVITY_THRESH]
  S1 -> S2 [commented out] : [ADAPTED_RATE == MAX_SENSE]
  S4 -> S3 [order 3] : [ADAPTED_RATE >= TARGET_RATE]
  Start -> S1 [commented out] : [ACTIVITY >= ACTIVITY_THRESH]
  Start1 -> S4 [order 1] : [ACTIVITY >= ACTIVITY_THRESH]
  Start1 -> Start1 [order 2] : [ACTIVITY < ACTIVITY_THRESH]
  S2FAIL -> Start [commented out] : [ADAPTED_RATE == LOWER_RATE_LIMIT]
  S2 -> S2FAIL [commented out] : [ACTIVITY < ACTIVITY_THRESH]
  S3 -> S2FAIL1 [order 1] : [ACTIVITY < ACTIVITY_THRESH]
  S_FAILSAFE -> S1 [commented out] : [ACTIVITY >= ACTIVITY_THRESH]
  S1 -> S_FAILSAFE [commented out] : [ACTIVITY <  ACTIVITY_THRESH]
  S2FAIL -> S1 [commented out] : [ACTIVITY >= ACTIVITY_THRESH]
  S4 -> S_FAILSAFE1 [order 2] : [ACTIVITY <  ACTIVITY_THRESH]
  S_FAILSAFE1 -> S4 [order 1] : [ACTIVITY >= ACTIVITY_THRESH]
  S2FAIL1 -> S4 [order 3] : [ACTIVITY >= ACTIVITY_THRESH]
  S2FAIL1 -> Start1 [order 1] : [ADAPTED_RATE <= LOWER_RATE_LIMIT]
  S_FAILSAFE1 -> S2FAIL1 [order 2] : [ after(1000,msec)]
  S_FAILSAFE -> S2FAIL [commented out] : [after(1000,msec)]
  S2FAIL -> S2FAIL [commented out] : after(1000, msec)[ADAPTED_RATE ~= LOWER_RATE_LIMIT]
  S2FAIL1 -> S2FAIL1 [order 2] : after(1000, msec)[ADAPTED_RATE >= LOWER_RATE_LIMIT]
  data: ACTIVITY input; ADAPTED_RATE output uint16; MAX_SENSE input uint16; REACT_TIME input uint16; RESP_FACTOR input; ACTIVITY_THRESH input double; RCVR_TIME input uint16; LOWER_RATE_LIMIT input uint16; step_up local uint16; step_down local uint16; TARGET_RATE input uint16
